simulink library "SIXOSEM_F_STAGE_MASTER"  (Simulink 8.6)
settings: Solver=ode45  StartTime=0.0  StopTime=10.0  RelTol=1e-3
libraries: cdsEpicsOut x196, cdsFilt x125, cdsTP x84, cdsFiltCtrl x37, cdsEpicsIn x36, cdsMuxMatrix x23, VIS_LIB x12, cdsEpicsBinIn x8, lockin x8, SIXOSEM_F_COILOUTF_MASTER x4, rtdemod x4, cdsOsc x4
(part 2 of 17)

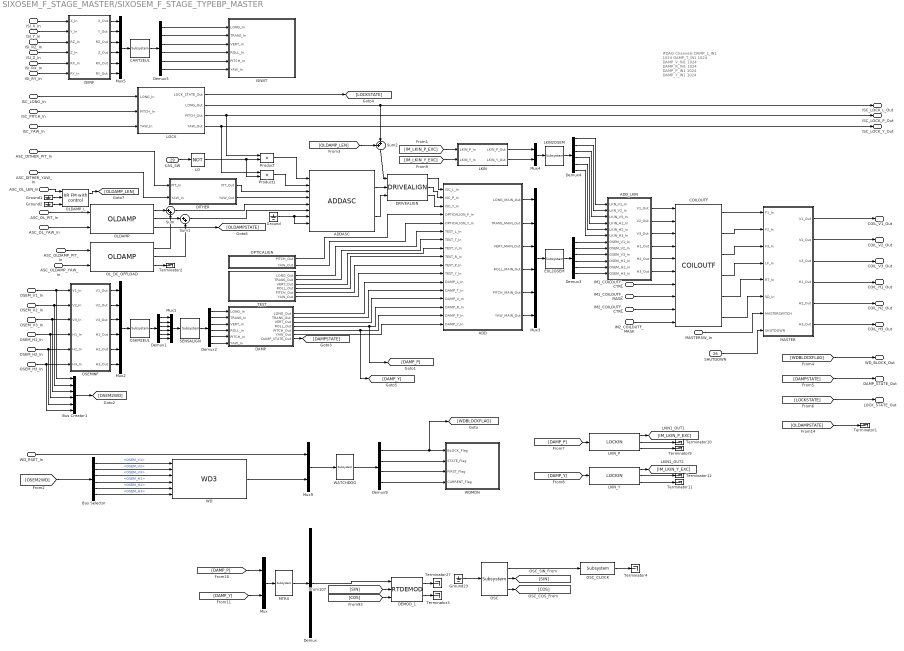
== system SIXOSEM_F_STAGE_MASTER/SIXOSEM_F_STAGE_TYPEBP_MASTER ==
  note: #DAQ Channels
      | DAMP_L_IN1 1024
      | DAMP_T_IN1 1024
      | DAMP_V_IN1 1024
      | DAMP_R_IN1 1024
      | DAMP_P_IN1 1024
      | DAMP_Y_IN1 1024
  ISI_X_In : Inport
  ISI_Y_In : Inport  Port=2
  ISI_RZ_In : Inport  Port=3
  ISI_Z_In : Inport  Port=4
  ISI_RX_In : Inport  Port=5
  ISI_RY_In : Inport  Port=6
  OSEM_V1_In : Inport  Port=7
  OSEM_V2_In : Inport  Port=8
  OSEM_V3_In : Inport  Port=9
  OSEM_H1_In : Inport  Port=10
  OSEM_H2_In : Inport  Port=11
  OSEM_H3_In : Inport  Port=12
  ISC_LONG_In : Inport  Port=13
  ISC_PITCH_In : Inport  Port=14
  ISC_YAW_In : Inport  Port=15
  ASC_DITHER_PIT_In : Inport  Port=16
  ASC_DITHER_YAW_In : Inport  Port=17
  IM1_COILOUTF_CTRL : Inport  Port=18
  IM1_COILOUTF_MASK : Inport  Port=19
  IM2_COILOUTF_CTRL : Inport  Port=20
  IM2_COILOUTF_MASK : Inport  Port=21
  MASTERSW_In : Inport  Port=22
  WD_RSET_In : Inport  Port=23
  ASC_OL_PIT_In : Inport  Port=24
  ASC_OL_YAW_In : Inport  Port=25
  SHUTDOWN : Inport  Port=26
  ASC_OLDAMP_PIT_In : Inport  Port=27
  ASC_OLDAMP_YAW_In : Inport  Port=28
  CAS_SW : Inport  Port=29
  ASC_OL_LEN_In : Inport  Port=30
  ADD : Subsystem
  ADDASC : VIS_LIB/ADDASC
  ADD_LKIN : Subsystem
  Bus Creator1 : BusCreator  Inputs='OSEM_V1','OSEM_V2','OSEM_V3','OSEM_H1','OSEM_H2','OSEM_H3'
  Bus Selector : BusSelector  OutputSignals=OSEM_V1,OSEM_V2,OSEM_V3,OSEM_H1,OSEM_H2,OSEM_H3
  CART2EUL : cdsMuxMatrix/Subsystem  Tag=cdsMuxMatrix  Description=Any size matrix. Inputs and outputs must be connected using Mux and Demux parts.
      settings: AttributesFormatString=%<Tag>
  COILOUTF : SIXOSEM_F_COILOUTF_MASTER/COILOUTF
  DAMP : Subsystem
  DEMOD_1 : rtdemod/RTDEMOD  Tag=top_names
  DITHER : Subsystem
  DRIVEALIGN : VIS_LIB/DRIVEALIGN
  Demux : Demux  Outputs=1
  Demux{1..5} (5 alike) : Demux  Outputs=6
  Demux9 : Demux
  EUL2OSEM : cdsMuxMatrix/Subsystem  Tag=cdsMuxMatrix  Description=Any size matrix. Inputs and outputs must be connected using Mux and Demux parts.
      settings: AttributesFormatString=%<Tag>
  Ground{,1..2,23} (4 alike) : Ground
  ISIINF : Subsystem
  ISIWIT : Subsystem
  LKIN : Subsystem
  LKIN2OSEM : cdsMuxMatrix/Subsystem  Tag=cdsMuxMatrix  Description=Any size matrix. Inputs and outputs must be connected using Mux and Demux parts.
      settings: AttributesFormatString=%<Tag>
  LKIN_P : lockin/LOCKIN  Description=ADL=LOCKIN.adl
      settings: AttributesFormatString=%<Tag>
  LKIN_Y : lockin/LOCKIN  Description=ADL=LOCKIN.adl
      settings: AttributesFormatString=%<Tag>
  LO : Logic  Operator=NOT  Inputs=1  AllPortsSameDT=off  OutDataTypeStr=boolean
  LOCK : Subsystem
  MASTER : Subsystem
  MTRX : cdsMuxMatrix/Subsystem  Tag=cdsMuxMatrix  Description=Any size matrix. Inputs and outputs must be connected using Mux and Demux parts.
      settings: AttributesFormatString=%<Tag>
  Mux : Mux  Inputs=2
  Mux{1..3,5} (4 alike) : Mux  Inputs=6
  Mux4 : Mux  Inputs=2
  Mux9 : Mux  Inputs=2
  OLDAMP : VIS_LIB/OLDAMP
  OLDAMP_L : cdsFiltCtrl/IIR FM with control  Tag=cdsFiltCtrl  Description=|
      | cdsFiltCntrl is the standard IIR filter module (exactly the same as cdsFilt) but with added control data output 'Ctrl'. Filter module digital signal output appears on the first output, which is called 'Val'. 'Ctrl' output has a bit pattern encoding the state of filter's on/off switches (FM1 through FM10). The bit values are:
      |                                                                                                                                                                                                                                                                                                                                       
      | module 	hex	dec                                                                                                                                                                                                                                                                                                                       
      | -----------------------                                                                                                                                                                                                                                                                                                               
      | FM1	0x20                    32                                                                                                                                                                                                                                                                                                        
      | FM2	0x80                     128                                                                                                                                                                                                                                                                                                      
      | FM3	0x200                   512                                                                                                                                                                                                                                                                                                       
      | FM4	0x800                   2048                                                                                                                                                                                                                                                                                                      
      | FM5	0x2000                 8192                                                                                                                                                                                                                                                                                                       
      | FM6	0x8000                 32768                                                                                                                                                                                                                                                                                                      
      | FM7	0x20000                131072                                                                                                                                                                                                                                                                                                     
      | FM8	0x80000                 524288                                                                                                                                                                                                                                                                                                    
      | FM9	0x200000               2097152                                                                                                                                                                                                                                                                                                    
      | FM10	0x800000               8388608                                                                                                                                                                                                                                                                                                   
      |                                                                                                                                                                                                                                                                                                                                       
      | This bit data can be used to drive some other switches or it can be output using a binary I/O module.
      settings: AttributesFormatString=%<Tag>
  OL_DC_OFFLOAD : VIS_LIB/OLDAMP
  OPTICALIGN : Subsystem
  OSC : cdsOsc/Subsystem  Tag=cdsOsc  Description=Oscillator
      settings: AttributesFormatString=%<Tag>
  OSC_CLOCK : cdsEpicsOut/Subsystem  Tag=cdsEpicsOutput  Description=|
      | Purpose:                                          
      | Output a FE signal to an EPICS channel.           
      |                                                   
      | Operation:                                        
      | Takes input value and passes it to EPICS record.  
      |                                                   
      | Usage:                                            
      | Name the part with the desired EPICS rrecord name.
      settings: AttributesFormatString=%<Tag>
  OSEM2EUL : cdsMuxMatrix/Subsystem  Tag=cdsMuxMatrix  Description=Any size matrix. Inputs and outputs must be connected using Mux and Demux parts.
      settings: AttributesFormatString=%<Tag>
  OSEMINF : Subsystem
  Product : Product
  Product1 : Product
  SENSALIGN : cdsMuxMatrix/Subsystem  Tag=cdsMuxMatrix  Description=Any size matrix. Inputs and outputs must be connected using Mux and Demux parts.
      settings: AttributesFormatString=%<Tag>
  Sum : Sum  Inputs=|++
  Sum1 : Sum  Inputs=|++
  Sum2 : Sum  Inputs=++|
  TEST : Subsystem
  Terminator{1..4,9..12,27} (9 alike) : Terminator
  WATCHDOG : cdsFunctionCall/Subsystem  Tag=cdsFunctionCall  Description=inline OSEMWATCHDOG /opt/rtcds/userapps/release/vis/common/src/WATCHDOG.c
      settings: AttributesFormatString=%<Tag>\n%<Description>
  WD : VIS_LIB/WD3
  WDMON : Subsystem
  ISC_LOCK_L_Out : Outport
  ISC_LOCK_P_Out : Outport  Port=2
  ISC_LOCK_Y_Out : Outport  Port=3
  COIL_V1_Out : Outport  Port=4
  COIL_V2_Out : Outport  Port=5
  COIL_V3_Out : Outport  Port=6
  COIL_H1_Out : Outport  Port=7
  COIL_H2_Out : Outport  Port=8
  COIL_H3_Out : Outport  Port=9
  WD_BLOCK_Out : Outport  Port=10
  DAMP_STATE_Out : Outport  Port=11
  LOCK_STATE_Out : Outport  Port=12
  wires:
  WATCHDOG/1 -> Demux9/1
  Mux9/1 -> WATCHDOG/1
  COILOUTF/6 -> MASTER/6(SD_In)
  COILOUTF/5 -> MASTER/5(RT_In)
  COILOUTF/4 -> MASTER/4(LF_In)
  COILOUTF/3 -> MASTER/3(F3_In)
  COILOUTF/2 -> MASTER/2(F2_In)
  COILOUTF/1 -> MASTER/1(F1_In)
  Demux9/4 -> WDMON/4(CURRENT_Flag)
  Demux9/3 -> WDMON/3(FIRST_Flag)
  Demux9/2 -> WDMON/2(STATE_Flag)
  Demux9/1 -> WDMON/1(BLOCK_Flag), [WDBLOCKFLAG]
  EUL2OSEM/1 -> Demux3/1
  Mux3/1 -> EUL2OSEM/1
  MASTER/6(H3_Out) -> COIL_H3_Out/1
  MASTER/5(H2_Out) -> COIL_H2_Out/1
  MASTER/4(H1_Out) -> COIL_H1_Out/1
  MASTER/3(V3_Out) -> COIL_V3_Out/1
  MASTER/2(V2_Out) -> COIL_V2_Out/1
  MASTER/1(V1_Out) -> COIL_V1_Out/1
  SENSALIGN/1 -> Demux2/1
  Mux1/1 -> SENSALIGN/1
  Demux1/6 -> Mux1/6
  Demux1/5 -> Mux1/5
  Demux1/4 -> Mux1/4
  Demux1/3 -> Mux1/3
  Demux1/2 -> Mux1/2
  Demux1/1 -> Mux1/1
  OSEM2EUL/1 -> Demux1/1
  Bus Selector/6 -> WD/6  "<OSEM_H3>"
  Bus Selector/5 -> WD/5  "<OSEM_H2>"
  Bus Selector/4 -> WD/4  "<OSEM_H1>"
  Bus Selector/3 -> WD/3  "<OSEM_V3>"
  Bus Selector/2 -> WD/2  "<OSEM_V2>"
  Bus Selector/1 -> WD/1  "<OSEM_V1>"
  [OSEM2WD] -> Bus Selector/1
  Bus Creator1/1 -> [OSEM2WD]
  ISC_YAW_In/1 -> LOCK/3(YAW_In)
  ISC_PITCH_In/1 -> LOCK/2(PITCH_In)
  ISC_LONG_In/1 -> LOCK/1(LONG_In)
  Mux2/1 -> OSEM2EUL/1
  OSEM_H3_In/1 -> Bus Creator1/6, OSEMINF/6(H3_In)
  OSEM_H2_In/1 -> Bus Creator1/5, OSEMINF/5(H2_In)
  OSEM_H1_In/1 -> Bus Creator1/4, OSEMINF/4(H1_In)
  OSEM_V3_In/1 -> Bus Creator1/3, OSEMINF/3(V3_In)
  OSEM_V2_In/1 -> Bus Creator1/2, OSEMINF/2(V2_In)
  OSEM_V1_In/1 -> Bus Creator1/1, OSEMINF/1(V1_In)
  OSEMINF/1(V1_Out) -> Mux2/1
  OSEMINF/2(V2_Out) -> Mux2/2
  OSEMINF/3(V3_Out) -> Mux2/3
  OSEMINF/4(H1_Out) -> Mux2/4
  OSEMINF/5(H2_Out) -> Mux2/5
  OSEMINF/6(H3_Out) -> Mux2/6
  ISI_X_In/1 -> ISIINF/1(X_In)
  ISI_Y_In/1 -> ISIINF/2(Y_In)
  ISI_RZ_In/1 -> ISIINF/3(RZ_In)
  ISI_Z_In/1 -> ISIINF/4(Z_In)
  ISI_RX_In/1 -> ISIINF/5(RX_In)
  ISI_RY_In/1 -> ISIINF/6(RY_In)
  ISIINF/1(X_Out) -> Mux5/1
  ISIINF/2(Y_Out) -> Mux5/2
  ISIINF/3(RZ_Out) -> Mux5/3
  ISIINF/4(Z_Out) -> Mux5/4
  ISIINF/5(RX_Out) -> Mux5/5
  ISIINF/6(RY_Out) -> Mux5/6
  Mux5/1 -> CART2EUL/1
  CART2EUL/1 -> Demux5/1
  Demux5/1 -> ISIWIT/1(LONG_In)
  Demux5/2 -> ISIWIT/2(TRANS_In)
  Demux5/3 -> ISIWIT/3(VERT_In)
  Demux5/4 -> ISIWIT/4(ROLL_In)
  Demux5/5 -> ISIWIT/5(PITCH_In)
  Demux5/6 -> ISIWIT/6(YAW_In)
  SHUTDOWN/1 -> MASTER/8(SHUTDOWN)
  Demux2/1 -> DAMP/1(LONG_In)
  Demux2/2 -> DAMP/2(TRANS_In)
  Demux2/3 -> DAMP/3(VERT_In)
  Demux2/4 -> DAMP/4(ROLL_In)
  Demux2/5 -> DAMP/5(PITCH_In)
  Demux2/6 -> DAMP/6(YAW_In)
  [WDBLOCKFLAG] -> WD_BLOCK_Out/1
  DAMP/7(DAMP_STATE_Out) -> [DAMPSTATE]
  [DAMPSTATE] -> DAMP_STATE_Out/1
  ADD/1(LONG_MAIN_Out) -> Mux3/1
  ADD/2(TRANS_MAIN_Out) -> Mux3/2
  ADD/3(VERT_MAIN_Out) -> Mux3/3
  ADD/4(ROLL_MAIN_Out) -> Mux3/4
  ADD/5(PITCH_MAIN_Out) -> Mux3/5
  ADD/6(YAW_MAIN_Out) -> Mux3/6
  LOCK/1(LOCK_STATE_Out) -> [LOCKSTATE]
  [LOCKSTATE] -> LOCK_STATE_Out/1
  LKIN/1(LKIN_P_Out) -> Mux4/1
  LKIN2OSEM/1 -> Demux4/1
  Mux4/1 -> LKIN2OSEM/1
  ADD_LKIN/1(V1_Out) -> COILOUTF/1
  ADD_LKIN/2(V2_Out) -> COILOUTF/2
  ADD_LKIN/3(V3_Out) -> COILOUTF/3
  ADD_LKIN/4(H1_Out) -> COILOUTF/4
  ADD_LKIN/5(H2_Out) -> COILOUTF/5
  ADD_LKIN/6(H3_Out) -> COILOUTF/6
  Demux4/1 -> ADD_LKIN/1(LKN_V1_In)
  Demux4/2 -> ADD_LKIN/2(LKN_V2_In)
  Demux4/3 -> ADD_LKIN/3(LKIN_V3_In)
  Demux4/4 -> ADD_LKIN/4(LKIN_H1_In)
  Demux4/5 -> ADD_LKIN/5(LKIN_H2_In)
  Demux4/6 -> ADD_LKIN/6(LKIN_H3_In)
  Demux3/1 -> ADD_LKIN/7(OSEM_V1_In)
  Demux3/2 -> ADD_LKIN/8(OSEM_V2_In)
  Demux3/3 -> ADD_LKIN/9(OSEM_V3_In)
  Demux3/4 -> ADD_LKIN/10(OSEM_H1_In)
  Demux3/5 -> ADD_LKIN/11(OSEM_H2_In)
  Demux3/6 -> ADD_LKIN/12(OSEM_H3_In)
  MASTERSW_In/1 -> MASTER/7(MASTERSWITCH)
  IM1_COILOUTF_MASK/1 -> COILOUTF/8
  IM1_COILOUTF_CTRL/1 -> COILOUTF/7
  LKIN/2(LKIN_Y_Out) -> Mux4/2
  WD/1 -> Mux9/2
  WD_RSET_In/1 -> Mux9/1
  LOCK/2(LONG_Out) -> Sum2/2, ISC_LOCK_L_Out/1
  LOCK/3(PITCH_Out) -> Product/1, ISC_LOCK_P_Out/1
  LOCK/4(YAW_Out) -> Product1/1, ISC_LOCK_Y_Out/1
  DRIVEALIGN/3 -> ADD/3(ISC_Y_In)
  DRIVEALIGN/2 -> ADD/2(ISC_P_In)
  DRIVEALIGN/1 -> ADD/1(ISC_L_In)
  ADDASC/1 -> DRIVEALIGN/2
  ADDASC/2 -> DRIVEALIGN/3
  ASC_DITHER_YAW_In/1 -> DITHER/2(YAW_In)
  ASC_DITHER_PIT_In/1 -> DITHER/1(PIT_In)
  DITHER/2(YAW_Out) -> ADDASC/4
  DITHER/1(PIT_Out) -> ADDASC/3
  OPTICALIGN/2(YAW_Out) -> ADD/5(OPTICALIGN_Y_In)
  OPTICALIGN/1(PITCH_Out) -> ADD/4(OPTICALIGN_P_In)
  TEST/6(YAW_Out) -> ADD/11(TEST_Y_In)
  TEST/5(PITCH_Out) -> ADD/10(TEST_P_In)
  TEST/4(ROLL_Out) -> ADD/9(TEST_R_In)
  TEST/3(VERT_Out) -> ADD/8(TEST_V_In)
  TEST/2(TRANS_Out) -> ADD/7(TEST_T_In)
  TEST/1(LONG_Out) -> ADD/6(TEST_L_In)
  DAMP/6(YAW_Out) -> ADD/17(DAMP_Y_In)
  DAMP/5(PITCH_Out) -> [DAMP_Y], ADD/16(DAMP_P_In)
  DAMP/4(ROLL_Out) -> [DAMP_P], ADD/15(DAMP_R_In)
  DAMP/3(VERT_Out) -> ADD/14(DAMP_V_In)
  DAMP/2(TRANS_Out) -> ADD/13(DAMP_T_In)
  DAMP/1(LONG_Out) -> ADD/12(DAMP_L_In)
  LKIN_P/2 -> Terminator10/1
  LKIN_P/3 -> Terminator9/1
  LKIN_P/1 -> [IM_LKIN_P_EXC]
  LKIN_Y/1 -> [IM_LKIN_Y_EXC]
  LKIN_Y/2 -> Terminator12/1
  LKIN_Y/3 -> Terminator11/1
  [IM_LKIN_P_EXC] -> LKIN/1(LKIN_P_In)
  [IM_LKIN_Y_EXC] -> LKIN/2(LKIN_Y_In)
  [DAMP_P] -> LKIN_P/1
  [DAMP_Y] -> LKIN_Y/1
  [DAMP_Y] -> Mux/2
  [DAMP_P] -> Mux/1
  OSC/3 -> [COS]
  OSC/2 -> [SIN]
  OSC_CLOCK/1 -> Terminator4/1
  OSC/1 -> OSC_CLOCK/1
  Ground23/1 -> OSC/1
  DEMOD_1/2 -> Terminator3/1
  DEMOD_1/1 -> Terminator27/1
  [COS] -> DEMOD_1/3
  [SIN] -> DEMOD_1/2
  Demux/1 -> DEMOD_1/1
  MTRX/1 -> Demux/1
  Mux/1 -> MTRX/1
  OLDAMP/3 -> [OLDAMPSTATE]
  ASC_OL_YAW_In/1 -> OLDAMP/2
  ASC_OL_PIT_In/1 -> OLDAMP/1
  [OLDAMPSTATE] -> Terminator1/1
  IM2_COILOUTF_CTRL/1 -> COILOUTF/9
  IM2_COILOUTF_MASK/1 -> COILOUTF/10
  ASC_OLDAMP_YAW_In/1 -> OL_DC_OFFLOAD/2
  ASC_OLDAMP_PIT_In/1 -> OL_DC_OFFLOAD/1
  OL_DC_OFFLOAD/3 -> Terminator2/1
  OLDAMP/1 -> Sum/1
  OL_DC_OFFLOAD/1 -> Sum/2
  Sum/1 -> ADDASC/5
  OLDAMP/2 -> Sum1/1
  Sum1/1 -> ADDASC/6
  OL_DC_OFFLOAD/2 -> Sum1/2
  Product/1 -> ADDASC/1
  Product1/1 -> ADDASC/2
  LO/1 -> Product1/2, Product/2
  CAS_SW/1 -> LO/1
  Ground/1 -> ADDASC/8, ADDASC/7
  ASC_OL_LEN_In/1 -> OLDAMP_L/1
  OLDAMP_L/1 -> [OLDAMP_LEN]
  [OLDAMP_LEN] -> Sum2/1
  Sum2/1 -> DRIVEALIGN/1
  Ground2/1 -> OLDAMP_L/3
  Ground1/1 -> OLDAMP_L/2

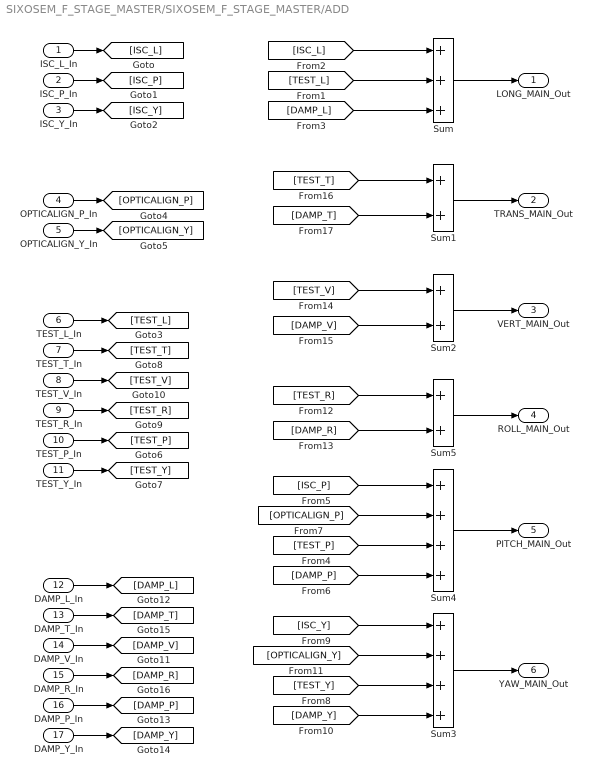
== system SIXOSEM_F_STAGE_MASTER/SIXOSEM_F_STAGE_MASTER/ADD ==
  ISC_L_In : Inport
  ISC_P_In : Inport  Port=2
  ISC_Y_In : Inport  Port=3
  OPTICALIGN_P_In : Inport  Port=4
  OPTICALIGN_Y_In : Inport  Port=5
  TEST_L_In : Inport  Port=6
  TEST_T_In : Inport  Port=7
  TEST_V_In : Inport  Port=8
  TEST_R_In : Inport  Port=9
  TEST_P_In : Inport  Port=10
  TEST_Y_In : Inport  Port=11
  DAMP_L_In : Inport  Port=12
  DAMP_T_In : Inport  Port=13
  DAMP_V_In : Inport  Port=14
  DAMP_R_In : Inport  Port=15
  DAMP_P_In : Inport  Port=16
  DAMP_Y_In : Inport  Port=17
  Sum : Sum  Inputs=+++
  Sum1 : Sum
  Sum2 : Sum
  Sum3 : Sum  Inputs=++++
  Sum4 : Sum  Inputs=++++
  Sum5 : Sum
  LONG_MAIN_Out : Outport
  TRANS_MAIN_Out : Outport  Port=2
  VERT_MAIN_Out : Outport  Port=3
  ROLL_MAIN_Out : Outport  Port=4
  PITCH_MAIN_Out : Outport  Port=5
  YAW_MAIN_Out : Outport  Port=6
  wires:
  Sum4/1 -> PITCH_MAIN_Out/1
  Sum3/1 -> YAW_MAIN_Out/1
  Sum/1 -> LONG_MAIN_Out/1
  [ISC_L] -> Sum/1
  [TEST_L] -> Sum/2
  [DAMP_L] -> Sum/3
  Sum5/1 -> ROLL_MAIN_Out/1
  Sum2/1 -> VERT_MAIN_Out/1
  Sum1/1 -> TRANS_MAIN_Out/1
  OPTICALIGN_P_In/1 -> [OPTICALIGN_P]
  OPTICALIGN_Y_In/1 -> [OPTICALIGN_Y]
  ISC_L_In/1 -> [ISC_L]
  ISC_P_In/1 -> [ISC_P]
  ISC_Y_In/1 -> [ISC_Y]
  TEST_L_In/1 -> [TEST_L]
  TEST_T_In/1 -> [TEST_T]
  TEST_V_In/1 -> [TEST_V]
  TEST_R_In/1 -> [TEST_R]
  TEST_P_In/1 -> [TEST_P]
  TEST_Y_In/1 -> [TEST_Y]
  DAMP_L_In/1 -> [DAMP_L]
  DAMP_T_In/1 -> [DAMP_T]
  DAMP_V_In/1 -> [DAMP_V]
  DAMP_R_In/1 -> [DAMP_R]
  DAMP_P_In/1 -> [DAMP_P]
  DAMP_Y_In/1 -> [DAMP_Y]
  [ISC_P] -> Sum4/1
  [OPTICALIGN_P] -> Sum4/2
  [TEST_P] -> Sum4/3
  [DAMP_P] -> Sum4/4
  [ISC_Y] -> Sum3/1
  [OPTICALIGN_Y] -> Sum3/2
  [TEST_Y] -> Sum3/3
  [DAMP_Y] -> Sum3/4
  [TEST_R] -> Sum5/1
  [DAMP_R] -> Sum5/2
  [TEST_T] -> Sum1/1
  [DAMP_T] -> Sum1/2
  [TEST_V] -> Sum2/1
  [DAMP_V] -> Sum2/2

== system SIXOSEM_F_STAGE_MASTER/SIXOSEM_F_STAGE_MASTER/ADDASC ==
  ISC_P_In : Inport
  ISC_Y_In : Inport  Port=2
  DITHER_P_In : Inport  Port=3
  DITHER_Y_In : Inport  Port=4
  OLDCCTRL_P_In : Inport  Port=5
  OLDCCTRL_Y_In : Inport  Port=6
  Sum3 : Sum  Inputs=+++
  Sum4 : Sum  Inputs=+++
  PITCH_Out : Outport
  YAW_Out : Outport  Port=2
  wires:
  Sum3/1 -> YAW_Out/1
  ISC_P_In/1 -> Sum4/1
  ISC_Y_In/1 -> Sum3/1
  Sum4/1 -> PITCH_Out/1
  DITHER_P_In/1 -> Sum4/2
  DITHER_Y_In/1 -> Sum3/2
  OLDCCTRL_P_In/1 -> Sum4/3
  OLDCCTRL_Y_In/1 -> Sum3/3

== system SIXOSEM_F_STAGE_MASTER/SIXOSEM_F_STAGE_MASTER/ADD_LKIN ==
  LKN_V1_In : Inport
  LKN_V2_In : Inport  Port=2
  LKIN_V3_In : Inport  Port=3
  LKIN_H1_In : Inport  Port=4
  LKIN_H2_In : Inport  Port=5
  LKIN_H3_In : Inport  Port=6
  OSEM_V1_In : Inport  Port=7
  OSEM_V2_In : Inport  Port=8
  OSEM_V3_In : Inport  Port=9
  OSEM_H1_In : Inport  Port=10
  OSEM_H2_In : Inport  Port=11
  OSEM_H3_In : Inport  Port=12
  Sum{,1..5} (6 alike) : Sum
  V1_Out : Outport
  V2_Out : Outport  Port=2
  V3_Out : Outport  Port=3
  H1_Out : Outport  Port=4
  H2_Out : Outport  Port=5
  H3_Out : Outport  Port=6
  wires:
  OSEM_H1_In/1 -> Sum1/2
  Sum1/1 -> H1_Out/1
  OSEM_V2_In/1 -> Sum4/2
  OSEM_V3_In/1 -> Sum3/2
  Sum4/1 -> V2_Out/1
  Sum3/1 -> V3_Out/1
  OSEM_V1_In/1 -> Sum/2
  LKN_V1_In/1 -> Sum/1
  Sum/1 -> V1_Out/1
  LKN_V2_In/1 -> Sum4/1
  LKIN_V3_In/1 -> Sum3/1
  LKIN_H1_In/1 -> Sum1/1
  OSEM_H3_In/1 -> Sum2/2
  Sum2/1 -> H3_Out/1
  OSEM_H2_In/1 -> Sum5/2
  Sum5/1 -> H2_Out/1
  LKIN_H2_In/1 -> Sum5/1
  LKIN_H3_In/1 -> Sum2/1
